simulink model "Model_Simulink_Proiect"  (R2023a)
settings: Solver=VariableStepAuto  StartTime=0.0  StopTime=100  RelTol=1e-3
undefined symbols (not defined in the file or in its folder): param
settings Model: Creator=Admin  LastModifiedBy=Admin

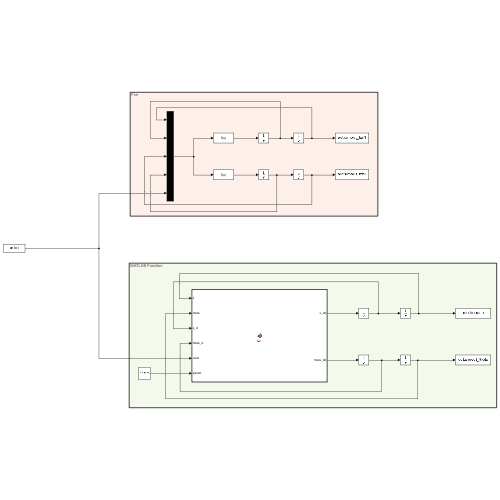
[thumbnail: Simulink's stored preview of the top-level diagram]
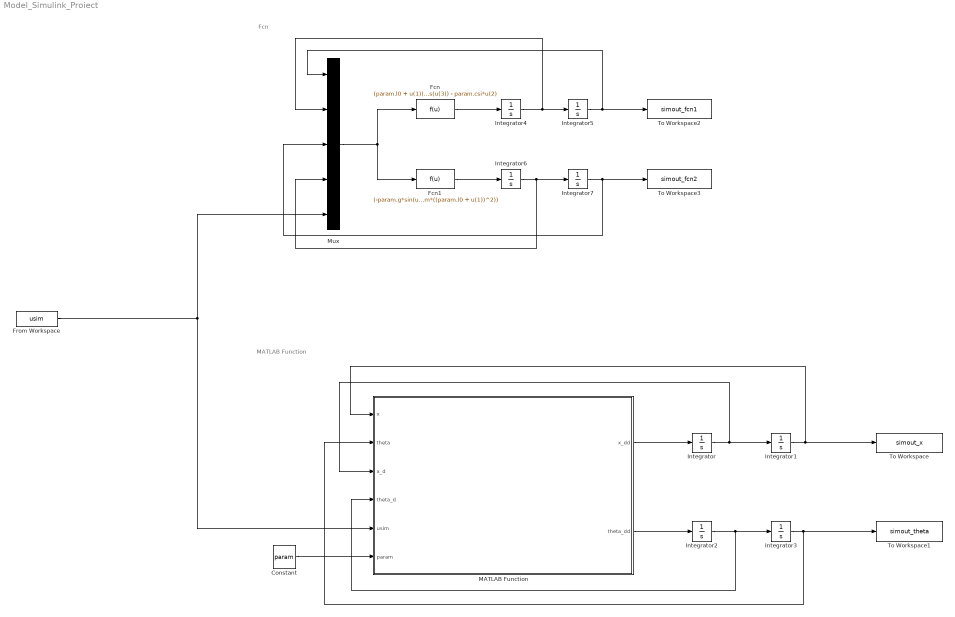
== system Model_Simulink_Proiect ==
  note: Fcn
  note: MATLAB Function
  Constant : Constant  Value=param  OutDataTypeStr=Bus: par_bus
  Fcn : Fcn  Expr=(param.l0 + u(1))*u(4)^2 - (param.k/param.m)*u(1) + param.g*cos(u(3)) - param.csi*u(2)
  Fcn1 : Fcn  Expr=(-param.g*sin(u(3)))/(param.l0 + u(1)) + (-2*u(2)*u(4))/(param.l0 + u(1)) - param.csi*u(4) + u(5)/(param.m*((param.l0 + u(1))^2))
  From Workspace : FromWorkspace  VariableName=usim
  Integrator{,1..7} (8 alike) : Integrator
  MATLAB Function : MATLAB Function  TreatAsAtomicUnit=on
  Mux : Mux  Inputs=5
  To Workspace : ToWorkspace  VariableName=simout_x  SaveFormat=Timeseries  SampleTime=-1
  To Workspace1 : ToWorkspace  VariableName=simout_theta  SaveFormat=Timeseries  SampleTime=-1
  To Workspace2 : ToWorkspace  VariableName=simout_fcn1  SaveFormat=Timeseries  SampleTime=-1
  To Workspace3 : ToWorkspace  VariableName=simout_fcn2  SaveFormat=Timeseries  SampleTime=-1
  wires:
  Constant/1 -> MATLAB Function/6(param)
  MATLAB Function/1(x_dd) -> Integrator/1
  MATLAB Function/2(theta_dd) -> Integrator2/1
  Integrator/1 -> Integrator1/1, MATLAB Function/3(x_d)
  Integrator2/1 -> Integrator3/1, MATLAB Function/4(theta_d)
  Integrator1/1 -> To Workspace/1, MATLAB Function/1(x)
  Integrator3/1 -> To Workspace1/1, MATLAB Function/2(theta)
  From Workspace/1 -> Mux/5, MATLAB Function/5(usim)
  Mux/1 -> Fcn1/1, Fcn/1
  Fcn/1 -> Integrator4/1
  Fcn1/1 -> Integrator6/1
  Integrator4/1 -> Integrator5/1, Mux/2
  Integrator6/1 -> Integrator7/1, Mux/4
  Integrator5/1 -> To Workspace2/1, Mux/1
  Integrator7/1 -> To Workspace3/1, Mux/3

== matlab function Model_Simulink_Proiect/MATLAB Function ==
  data: x input; x_dd output; theta input; x_d input; theta_d input; usim input; param input; theta_dd output
function [x_dd, theta_dd] = fcn(x, theta, x_d, theta_d, usim, param)
x_dd = (param.l0 + x)*theta_d^2 - (param.k/param.m)*x + param.g*cos(theta) - param.csi*x_d;
theta_dd = (-param.g/(param.l0 + x))*sin(theta) - ((2*x_d)/(param.l0 + x))*theta_d - param.csi*theta_d + usim/(param.m*((param.l0+x)^2)); 
end
